simulink model "untitled2"  (R2022a)
settings: Solver=VariableStepAuto  StartTime=0.0  StopTime=10.0  RelTol=1e-3
settings Model: Creator=mauricionakai  LastModifiedBy=mauricionakai

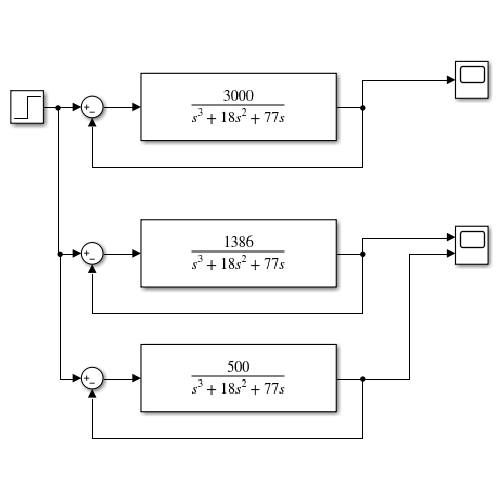
[thumbnail: Simulink's stored preview of the top-level diagram]
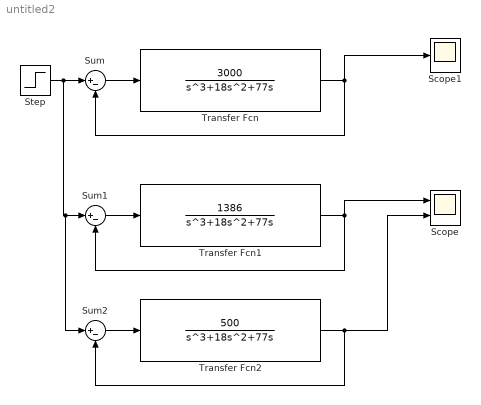
== system untitled2 ==
  Scope : Scope  NumInputPorts=2
  Scope1 : Scope
  Step : Step  SampleTime=0
  Sum : Sum  Inputs=|+-
  Sum1 : Sum  Inputs=|+-
  Sum2 : Sum  Inputs=|+-
  Transfer Fcn : TransferFcn  Numerator=[3000]  Denominator=[1 18 77 0]
  Transfer Fcn1 : TransferFcn  Numerator=[1386]  Denominator=[1 18 77 0]
  Transfer Fcn2 : TransferFcn  Numerator=[500]  Denominator=[1 18 77 0]
  wires:
  Sum/1 -> Transfer Fcn/1
  Transfer Fcn/1 -> Scope1/1, Sum/2
  Transfer Fcn1/1 -> Sum1/2, Scope/1
  Sum1/1 -> Transfer Fcn1/1
  Transfer Fcn2/1 -> Scope/2, Sum2/2
  Sum2/1 -> Transfer Fcn2/1
  Step/1 -> Sum2/1, Sum1/1, Sum/1
